simulink model "sf_tlafter"  (R2017b)
settings: Solver=ode45  StartTime=0.0  StopTime=100  RelTol=1e-3  EnableMultiTasking=on
settings Model: FPTRunName=Active  ExtModeAutoUpdateStatusClock=off  Creator=The MathWorks, Inc.  LastModifiedBy=The MathWorks, Inc.
settings DataIOCC: LimitDataPoints=on  SaveFormat=Array
settings OptimizationCC: BooleanDataType=off  ExpressionDepthLimit=2147483647  InitFltsAndDblsToZero=on  EfficientMapNaN2IntZero=off  LifeSpan=inf
settings DebuggingCC: SaveWithParameterizedLinksMsg=none  UnderspecifiedInitializationDetection=Classic  MergeDetectMultiDrivingBlocksExec=none  SignalResolutionControl=TryResolveAllWithWarning  MultiTaskDSMMsg=warning  MultiTaskCondExecSysMsg=none  FcnCallInpInsideContextMsg=warning  StateNameClashWarn=warning  StrictBusMsg=None  SFUnexpectedBacktrackingDiag=warning  SFNoUnconditionalDefaultTransitionDiag=warning  SFExecutionAtInitializationDiag=none
settings HardwareCC: ProdBitPerPointer=32  ProdBitPerSizeT=32  ProdBitPerPtrDiffT=32  ProdLargestAtomicFloat=None  ProdIntDivRoundTo=Undefined  ProdEndianess=Unspecified  ProdWordSize=32  ProdHWDeviceType=32-bit Generic  TargetUnknown=on
settings ModelReferenceCC: PropagateSignalLabelsOutOfModel=off
settings SFSimCC: SimParseCustomCode=off
settings CodeAppCC: StateflowObjectComments=on
settings GRTTargetCC: TargetFcnLib=ansi_tfl_tmw.mat  TargetLangStandard=C89/C90 (ANSI)  GeneratePreprocessorConditionals=Disable all  CombineOutputUpdateFcns=off  GRTInterface=on
settings ConfigComp: CovMetricSettings=dcmtr  CovHtmlReporting=on  CovSaveCumulativeToWorkspaceVar=on  CovSaveSingleToWorkspaceVar=on  CovExternalEMLEnable=off  CovSFcnEnable=off

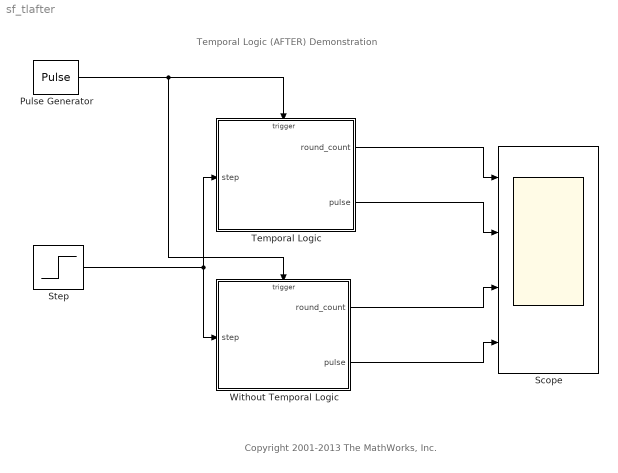
== system sf_tlafter ==
  note: Temporal Logic (AFTER) Demonstration
  note: Copyright 2001-2013 The MathWorks, Inc.
  Pulse Generator : DiscretePulseGenerator  PulseType=Time based  Period=1  PulseWidth=50
  Scope : Scope  NumInputPorts=4
  Step : Step  Time=60  SampleTime=0
  Temporal Logic : Stateflow chart  TreatAsAtomicUnit=on
  Without Temporal Logic : Stateflow chart  TreatAsAtomicUnit=on
  wires:
  Pulse Generator/1 -> Temporal Logic/Trigger, Without Temporal Logic/Trigger
  Temporal Logic/1(round_count) -> Scope/1
  Temporal Logic/2(pulse) -> Scope/2
  Without Temporal Logic/1(round_count) -> Scope/3
  Without Temporal Logic/2(pulse) -> Scope/4
  Step/1 -> Temporal Logic/1(step), Without Temporal Logic/1(step)

== stateflow chart sf_tlafter/Temporal Logic ==
  state Off
  state On
    en:pulse=1;
    exit:pulse=0;
  (default) -> Off : {round_count=0;}
  Off -> On : after(10,secs)[step<1]
  On -> Off : {round_count = round_count + 1;}
  data: round_count output double; pulse output double; step input double
  events: secs input RISING_EDGE_EVENT

== stateflow chart sf_tlafter/Without Temporal Logic ==
  state On [parallel]
    settings: executionOrder=1
    state B
      entry: pulse=1;
      exit: pulse=0;
    state A
      entry: count_after=2;
      A -> A [order 1] : {count_after = count_after + 1;}
    A -> B [order 1] : [count_after>10 && step<1]
    B -> A : {round_count = round_count + 1;}
  (default) -> A : {round_count =0;}
  data: round_count output double; count_after local double; pulse output double; step input double
  events: secs input RISING_EDGE_EVENT
